simulink model "Sim_PID_02"  (R2020b)
settings: Solver=FixedStepAuto  StartTime=0.0  StopTime=simtime  FixedStep=1e-4  RelTol=1e-3
InitFcn:
  | PID_startup
values from neighbouring files (symbols this model uses):
  BLS = a^2*(Bm + Bt) + Bg    (= 0.00020001)    [PID_startup.m]
  CF = 500    [PID_startup.m]
  JLS = a^2*(Jm+Jp) + Jg + Jl    (= 0.00110051)    [PID_startup.m]
  K = 1    [PID_startup.m]
  Kd = 5    [PID_startup.m]
  Ki = 2    [PID_startup.m]
  Km = 6.95e-3    (= 0.00695)    [PID_startup.m]
  Kp = 2    [PID_startup.m]
  L = 1.8e-3    (= 0.0018)    [PID_startup.m]
  R = 2    [PID_startup.m]
  Sg = 1    [PID_startup.m]
settings Model: Creator=miyaz  LastModifiedBy=miyaz

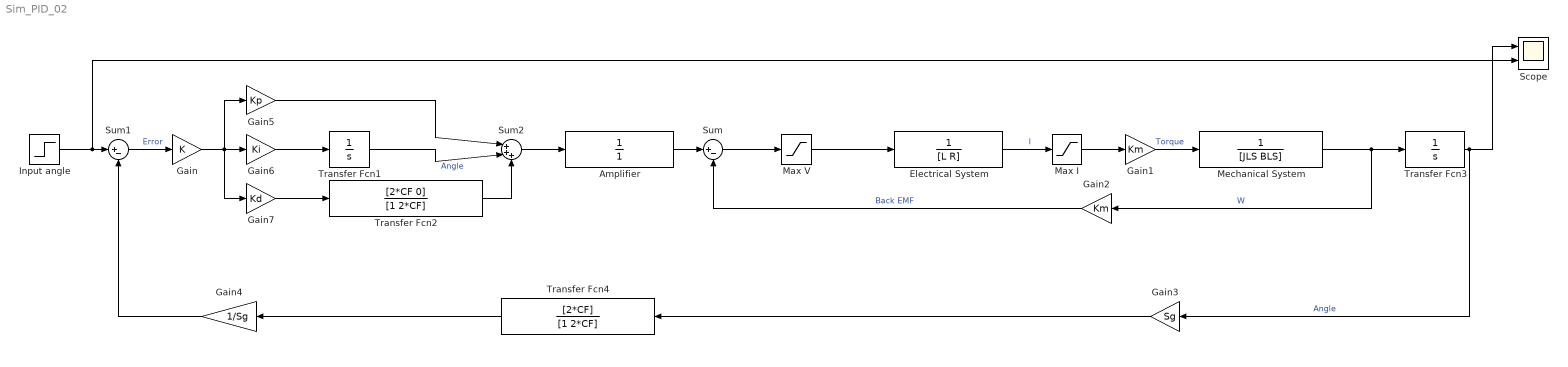
== system Sim_PID_02 ==
  Amplifier : TransferFcn  Denominator=[0 1]
  Electrical System : TransferFcn  Denominator=[L R]
  Gain : Gain  Gain=K
  Gain1 : Gain  Gain=Km
  Gain2 : Gain  Gain=Km
  Gain3 : Gain  Gain=Sg
  Gain4 : Gain  Gain=1/Sg
  Gain5 : Gain  Gain=Kp
  Gain6 : Gain  Gain=Ki
  Gain7 : Gain  Gain=Kd
  Input angle : Step  After=pi/2  SampleTime=0
  Max I : Saturate  UpperLimit=5  LowerLimit=-5
  Max V : Saturate  UpperLimit=50  LowerLimit=-50
  Mechanical System : TransferFcn  Denominator=[JLS BLS]
  Scope : Scope  NumInputPorts=2
  Sum : Sum  Inputs=|+-
  Sum1 : Sum  Inputs=|+-
  Sum2 : Sum  Inputs=|+++
  Transfer Fcn1 : TransferFcn  Denominator=[1 0]
  Transfer Fcn2 : TransferFcn  Numerator=[2*CF 0]  Denominator=[1 2*CF]
  Transfer Fcn3 : TransferFcn  Denominator=[1 0]
  Transfer Fcn4 : TransferFcn  Numerator=[2*CF]  Denominator=[1 2*CF]
  wires:
  Max V/1 -> Electrical System/1
  Max I/1 -> Gain1/1
  Amplifier/1 -> Sum/1
  Gain4/1 -> Sum1/2
  Sum/1 -> Max V/1
  Transfer Fcn4/1 -> Gain4/1
  Gain3/1 -> Transfer Fcn4/1
  Gain1/1 -> Mechanical System/1  "Torque"
  Transfer Fcn3/1 -> Gain3/1, Scope/1  "Angle"
  Gain2/1 -> Sum/2  "Back EMF"
  Mechanical System/1 -> Gain2/1, Transfer Fcn3/1  "W"
  Input angle/1 -> Sum1/1, Scope/2
  Sum1/1 -> Gain/1  "Error"
  Electrical System/1 -> Max I/1  "I"
  Gain5/1 -> Sum2/1
  Transfer Fcn1/1 -> Sum2/2  "Angle"
  Gain6/1 -> Transfer Fcn1/1
  Transfer Fcn2/1 -> Sum2/3
  Gain7/1 -> Transfer Fcn2/1
  Gain/1 -> Gain6/1, Gain5/1, Gain7/1
  Sum2/1 -> Amplifier/1
